simulink model "EV_Modeling"  (R2022a)
settings: Solver=FixedStepAuto  StartTime=0.0  StopTime=23612  FixedStep=0.1  RelTol=1e-3
values from neighbouring files (symbols this model uses):
  battery_SOC_SOC = battery_SOC(:,1)    [simulink.m]
  battery_SOC_voltage = battery_SOC(:,2)    [simulink.m]
  electric_consumption_ressistancce = electric_consumption(:,2)    [simulink.m]
  electric_consumption_voltage = electric_consumption(:,1)    [simulink.m]
  motor_efficiency_efficiency = table2array(motor_efficiency(2:height(motor_efficiency),2:width(motor_efficiency)))    [simulink.m]
  motor_efficiency_RPM = table2array(motor_efficiency(2:height(motor_efficiency),1))    [simulink.m]
  motor_efficiency_torque = transpose(motor_efficiency_torque)    [simulink.m]
  motor_RPM_torque = table2array(motor_torque(1:14,1))    [simulink.m]
  motor_torque_RPM = table2array(motor_torque(1:14,2))    [simulink.m]
libraries: simulink x4, simulink_extras x1, slpidlib x1
settings Model: Creator=Administrator  LastModifiedBy=jm538
settings SolverCC: AlgebraicLoopSolver=TrustRegion
settings DataIOCC: ExternalInput=EV_ModelingScenario.getElement('Input')  LoadExternalInput=on
settings DebuggingCC: UnconnectedInputMsg=warning  UnconnectedOutputMsg=warning  UnconnectedLineMsg=warning  SFMachineParentedDataDiag=warning
settings RTWCC: DLArmComputeVersion=19.05

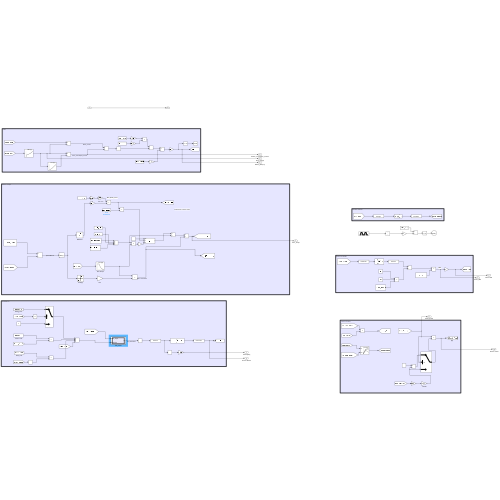
[thumbnail: Simulink's stored preview of the top-level diagram]
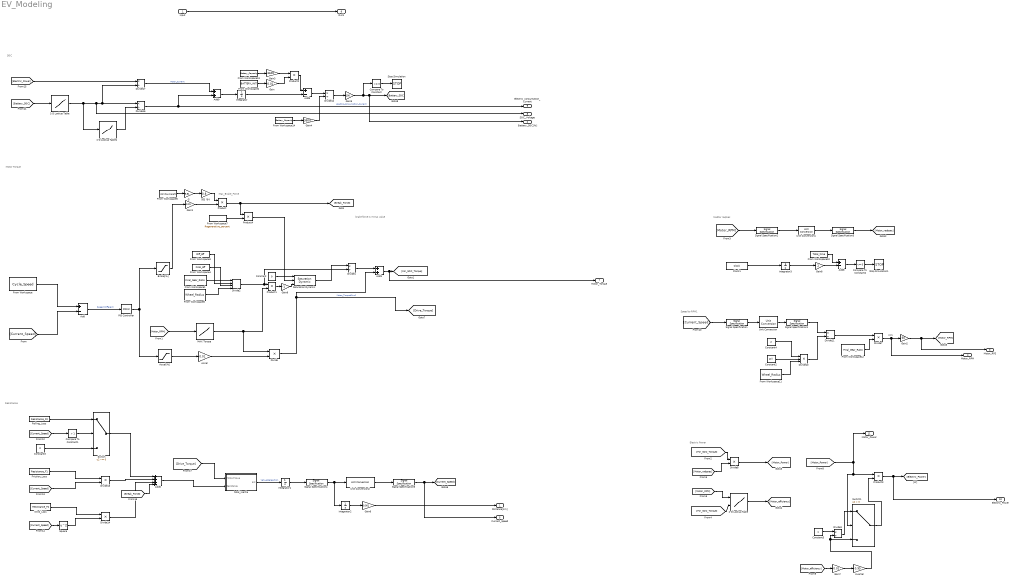
== system EV_Modeling ==
  note: brake force is minus value
  note: SOC
  note: Speed to RPM1
  note: Electric Power
  note: Resistance
  note: Motor Torque
  note: Modtor rad/sec
  note: Max_Brake_Force
  note: RPS
  Input : Inport
  1-D Lookup Table : Lookup_n-D  NumberOfTableDimensions=1  BreakpointsForDimension1=battery_SOC_SOC  Table=battery_SOC_voltage  InternalRulePriority=Speed  RndMeth=Simplest
  1-D Lookup Table1 : Lookup_n-D  NumberOfTableDimensions=1  BreakpointsForDimension1=electric_consumption_voltage  Table=electric_consumption_ressistancce  InternalRulePriority=Speed  RndMeth=Simplest
  2-D Lookup Table : Lookup_n-D  BreakpointsForDimension1=motor_efficiency_RPM  BreakpointsForDimension2=motor_efficiency_torque  Table=motor_efficiency_efficiency  InternalRulePriority=Speed  RndMeth=Simplest
      settings: InputPortMap=u0,u1
  Accel : Gain  Gain=0.01
  Accel[%] : Saturate  UpperLimit=100  LowerLimit=0
  Add : Sum  Inputs=+-
  Add1 : Sum
  Add5 : Sum  Inputs=+-
  Add6 : Sum  Inputs=+++-
  Add8 : Sum  Inputs=+-
  Add9 : Sum
  Brake[%] : Saturate  UpperLimit=0  LowerLimit=-100
  Clock1 : simulink_extras/Flip Flops/Clock  period=2
  Compare To Constant : simulink/Logic and Bit Operations/Compare To Constant  relop=<=  const=0  OutDataTypeStr=boolean
  Compare To Constant1 : simulink/Logic and Bit Operations/Compare To Constant  relop=>  const=1  OutDataTypeStr=boolean
  Compare To Constant2 : simulink/Logic and Bit Operations/Compare To Constant  relop=<=  const=0  OutDataTypeStr=boolean
  Constant : Constant  Value=0
  Constant2 : Constant  Value=pi()
  Constant3 : Constant  Value=0
  Constant4 : Constant  Value=2
  Constant5 : Constant
  Divide{,7..8,13..14} (5 alike) : Product  Inputs=**
  Divide{1,3,11..12,16..17} (6 alike) : Product  Inputs=*/
  Divide10 : Product  Inputs=***
  Divide2 : Product  Inputs=***/
  Friction_Loss : FromWorkspace  VariableName=Resistance_F1
  From Workspace : FromWorkspace  VariableName=Cycle_Speed
  From Workspace1 : FromWorkspace  VariableName=Final_Gear_Ratio
  From Workspace10 : FromWorkspace  VariableName=Total_time
  From Workspace11 : FromWorkspace  VariableName=Wheel_Radius
  From Workspace12 : FromWorkspace  VariableName=Final_Gear_Ratio
  From Workspace13 : FromWorkspace  VariableName=Battery_Capacity
  From Workspace14 : FromWorkspace  VariableName=Battery_Capacity
  From Workspace2 : FromWorkspace  VariableName=BATTERY_INIT
  From Workspace3 : FromWorkspace  VariableName=Diff_Eff
  From Workspace4 : FromWorkspace  VariableName=Final_Eff
  From Workspace5 : FromWorkspace  VariableName=Vehicle_Weight
  From Workspace6 : FromWorkspace  VariableName=Wheel_Radius
  From Workspace7 : FromWorkspace  VariableName=Regenerative_percent
  G : Gain  Gain=9.81
  Gain : Gain  Gain=0.01
  Gain1 : Gain  Gain=0.01
  Gain2 : Gain  Gain=60
  Gain3 : Gain  Gain=3600
  Gain4 : Gain  Gain=3600
  Gain5 : Gain  Gain=100
  Gain6 : Gain  Gain=0.001
  Gain7 : Gain  Gain=0.01
  Gain8 : Gain  Gain=2
  Gain9 : Gain  Gain=-1
  Integrator{,1..3} (4 alike) : Integrator
  MAX Torque : Lookup_n-D  NumberOfTableDimensions=1  BreakpointsForDimension1=motor_RPM_torque  Table=motor_torque_RPM  InternalRulePriority=Speed  RndMeth=Simplest
  PID Controller : slpidlib/PID Controller  Controller=PID  Form=Parallel  TimeDomain=Continuous-time  UseExternalTs=off  SampleTime=-1  IntegratorMethod=Forward Euler  FilterMethod=Forward Euler  ControllerParametersSource=internal  P=25  I=0.01  UseKiTs=off  D=0.0001  N=10  UseFilter=on  TunerSelectOption=Transfer Function Based (PID Tuner App)  InitialConditionSource=internal  InitialConditionForIntegrator=0  InitialConditionForFilter=0  DifferentiatorICPrevScaledInput=0  ExternalReset=none  TrackingMode=off  Kt=1  LimitOutput=off  SatLimitsSource=internal  UpperSaturationLimit=inf  LowerSaturationLimit=-inf  LinearizeAsGain=on  AntiWindupMode=none  Kb=1  POutMin=[]  POutMax=[]  IOutMin=[]  IOutMax=[]  DOutMin=[]  DOutMax=[]  NOutMin=[]  NOutMax=[]  SumOutMin=[]  SumOutMax=[]  SaturationOutMin=[]  SaturationOutMax=[]  PParamMin=[]  PParamMax=[]  IParamMin=[]  IParamMax=[]  DParamMin=[]  DParamMax=[]  NParamMin=[]  NParamMax=[]  KbParamMin=[]  KbParamMax=[]  KtParamMin=[]  KtParamMax=[]  KbOutMin=[]  KbOutMax=[]  KtOutMin=[]  KtOutMax=[]  IntegratorOutMin=[]  IntegratorOutMax=[]  FilterOutMin=[]  FilterOutMax=[]  SumI1OutMin=[]  SumI1OutMax=[]  SumI2OutMin=[]  SumI2OutMax=[]  SumI3OutMin=[]  SumI3OutMax=[]  SumI4OutMin=[]  SumI4OutMax=[]  SumDOutMin=[]  SumDOutMax=[]  DifferentiatorOutMin=[]  DifferentiatorOutMax=[]  FilterDiffOutCoefMin=[]  FilterDiffOutCoefMax=[]  ReciprocalOutMin=[]  ReciprocalOutMax=[]  SumDenOutMin=[]  SumDenOutMax=[]  SumNumOutMin=[]  SumNumOutMax=[]  DivideOutMin=[]  DivideOutMax=[]  UdiffTsProdOutMin=[]  UdiffTsProdOutMax=[]  NTsProdOutMin=[]  NTsProdOutMax=[]  UintegralTsProdOutMin=[]  UintegralTsProdOutMax=[]  UngainTsProdOutMin=[]  UngainTsProdOutMax=[]  IntegratorContinuousStateAttributes=''  IntegratorStateMustResolveToSignalObject=off  IntegratorRTWStateStorageClass=Auto  FilterContinuousStateAttributes=''  FilterStateMustResolveToSignalObject=off  FilterRTWStateStorageClass=Auto  ParallelPVariant=InternalParameters  IdealPVariant=Disabled  IVariant=InternalParameters  DVariant=InternalParameters  IntegratorVariant=Continuous  SatVariant=Disabled  AWVariant=Passthrough  PCopyVariant=Disabled  TRVariant=Disabled  FdbkBlocksVariant=Forward  IdealPFdbkVariant=Disabled  SatFdbkVariant=Disabled  DerivativeFilterVariant=ContFilter  NVariant=InternalParameters  NCopyVariant=Disabled  FilterICVariant=InternalICsFilter  IntegratorICVariant=InternalICs  ExternalResetVariant=Disabled  TRSumVariant=Passthrough  SumFdbkVariant=Disabled  SumVariant=Sum_PID  TsampFilterVariant=InternalTs  TsampNgainVariant=Passthrough  TsampIntegralVariant=Passthrough  ExternalSaturationOutDataTypeStr=Inherit: Same as second input  aMode=0
  Product{,1..4} (5 alike) : Product
  Rolling_Loss : FromWorkspace  VariableName=Resistance_F0
  Saturation Dynamic : simulink/Discontinuities/Saturation Dynamic  OutMin=[]  OutMax=[]  OutDataTypeStr=Inherit: Same as second input  OutDataType=fixdt(1, 16)  OutScaling=2^-10  DoSatur=off
  Signal Specification : SignalSpecification  Unit=km/hr
  Signal Specification1 : SignalSpecification  Unit=m/s
  Signal Specification2 : SignalSpecification  Unit=rpm
  Signal Specification3 : SignalSpecification  Unit=rad/s
  Signal Specification4 : SignalSpecification  Unit=m/s
  Signal Specification5 : SignalSpecification  Unit=km/hr
  Square : Math  Operator=square
  Stop Simulation : Stop
  Stop Simulation1 : Stop
  Switch : Switch  Criteria=u2 ~= 0  SaturateOnIntegerOverflow=off  InputSameDT=off
  Switch1 : Switch  Criteria=u2 > Threshold  SaturateOnIntegerOverflow=off  InputSameDT=off
  Unit Conversion : UnitConversion
  Unit Conversion1 : UnitConversion
  Unit Conversion2 : UnitConversion
  Wind_Loss : FromWorkspace  VariableName=Resistance_F2
  inverter : Gain  Gain=0.95
  total_inertia : Subsystem
  마찰 계수 : Gain  Gain=0.8
  Distance[km] : Outport
  Battery_SOC[%] : Outport  Port=2
  Motor_RPS : Outport  Port=3
  Motor_RPM : Outport  Port=4
  Current_Speed : Outport  Port=5
  Out1 : Outport  Port=6
  Motor_Torque : Outport  Port=7
  SOC_Voltage : Outport  Port=8
  Electric_consumption_Current : Outport  Port=9
  Electric_Power : Outport  Port=10
  Motor_Power : Outport  Port=11
  wires:
  Gain5/1 -> Battery_SOC[%]/1, [Battery_SOC], Compare To Constant/1
  1-D Lookup Table/1 -> Divide16/1, Divide17/2, SOC_Voltage/1, 1-D Lookup Table1/1
  Product3/1 -> Electric_Power/1, [Electric_Power]
  Gain6/1 -> Distance[km]/1
  Integrator3/1 -> Gain8/1
  Signal Specification5/1 -> Current_Speed/1, [Current_Speed]
  Compare To Constant2/1 -> Stop Simulation1/1
  Add8/1 -> Compare To Constant2/1
  Gain8/1 -> Add8/2
  From Workspace10/1 -> Add8/1
  Clock1/1 -> Integrator3/1
  Input/1 -> Out1/1
  Signal Specification2/1 -> Unit Conversion1/1
  Unit Conversion1/1 -> Signal Specification3/1
  Signal Specification3/1 -> [Motor_radpsec]
  Add1/1 -> Motor_Torque/1, [For_SOC_Torque]
  Divide1/1 -> Add1/1
  Divide2/1 -> Divide1/2, Product1/1
  From Workspace1/1 -> Divide2/1
  마찰 계수/1 -> Product/1
  G/1 -> 마찰 계수/1
  From Workspace5/1 -> G/1
  Accel/1 -> Divide/2
  Brake[%]/1 -> Gain1/1
  Divide/1 -> Add1/2, [Drive_Torque]  "Motor_Torque[N.m]"
  [Current_Speed] -> Add/2
  PID Controller/1 -> Brake[%]/1, Accel[%]/1
  Gain1/1 -> Product/2
  [Motor_RPM] -> MAX Torque/1
  MAX Torque/1 -> Product1/2, Divide/1
  From Workspace/1 -> Add/1
  Add/1 -> PID Controller/1  "Speed Different"
  Accel[%]/1 -> Accel/1
  [Current_Speed] -> Square/1
  Integrator2/1 -> Gain6/1
  Divide14/1 -> Add6/3
  Integrator1/1 -> Signal Specification4/1
  Wind_Loss/1 -> Divide14/1
  Signal Specification4/1 -> Integrator2/1, Unit Conversion2/1
  Unit Conversion2/1 -> Signal Specification5/1
  Rolling_Loss/1 -> Switch/1
  [Current_Speed] -> Divide13/2
  Square/1 -> Divide14/2
  total_inertia/1(acc) -> Integrator1/1  "Veh_acceleartion"
  [Current_Speed] -> Compare To Constant1/1
  Friction_Loss/1 -> Divide13/1
  Compare To Constant1/1 -> Switch/2
  Divide13/1 -> Add6/2
  Constant3/1 -> Switch/3
  Switch/1 -> Add6/1
  [Motor_RPM] -> Signal Specification2/1
  [Motor_efficiency] -> Gain7/1
  2-D Lookup Table/1 -> [Motor_efficiency]
  [For_SOC_Torque] -> Divide8/1
  [Motor_radpsec] -> Divide8/2
  Divide8/1 -> [Motor_Power]
  [For_SOC_Torque] -> 2-D Lookup Table/2
  [Motor_RPM] -> 2-D Lookup Table/1
  [Motor_Power] -> Motor_Power/1, Switch1/2, Product3/1
  From Workspace12/1 -> Divide7/2
  Constant4/1 -> Divide10/1
  Divide11/1 -> Divide7/1
  Constant2/1 -> Divide10/2
  Signal Specification1/1 -> Divide11/1
  [Current_Speed] -> Signal Specification/1
  From Workspace11/1 -> Divide10/3
  Signal Specification/1 -> Unit Conversion/1
  Gain2/1 -> Motor_RPS/1, [Motor_RPM]
  Divide10/1 -> Divide11/2
  Unit Conversion/1 -> Signal Specification1/1
  Divide7/1 -> Motor_RPM/1, Gain2/1
  Divide17/1 -> Add9/1  "Motor_Current"
  Divide12/1 -> Gain5/1
  From Workspace13/1 -> Gain3/1
  Divide16/1 -> Add9/2, Electric_consumption_Current/1  "electric_consumption_Current"
  From Workspace14/1 -> Gain4/1
  Integrator/1 -> Add5/2
  1-D Lookup Table1/1 -> Divide16/2
  [Battery_SOC] -> 1-D Lookup Table/1
  Compare To Constant/1 -> Stop Simulation/1
  Add5/1 -> Divide12/1
  Add9/1 -> Integrator/1
  [Electric_Power] -> Divide17/1
  Gain4/1 -> Divide12/2
  Product/1 -> [Break_Force], Product4/1
  [Drive_Torque] -> total_inertia/1(Motor_Toque)
  [Break_Force] -> Add6/4
  Add6/1 -> total_inertia/2(Resistance)
  From Workspace2/1 -> Gain/1
  Gain3/1 -> Product2/1
  Gain/1 -> Product2/2
  Product2/1 -> Add5/1
  Gain7/1 -> inverter/1
  Constant5/1 -> Divide3/1
  Switch1/1 -> Product3/2
  Divide3/1 -> Switch1/1
  From Workspace6/1 -> Divide2/4
  From Workspace4/1 -> Divide2/3
  From Workspace3/1 -> Divide2/2
  Product1/1 -> Gain9/1
  Gain9/1 -> Saturation Dynamic/3
  Constant/1 -> Saturation Dynamic/1
  Saturation Dynamic/1 -> Divide1/1
  From Workspace7/1 -> Product4/2
  Product4/1 -> Saturation Dynamic/2
  inverter/1 -> Divide3/2, Switch1/3

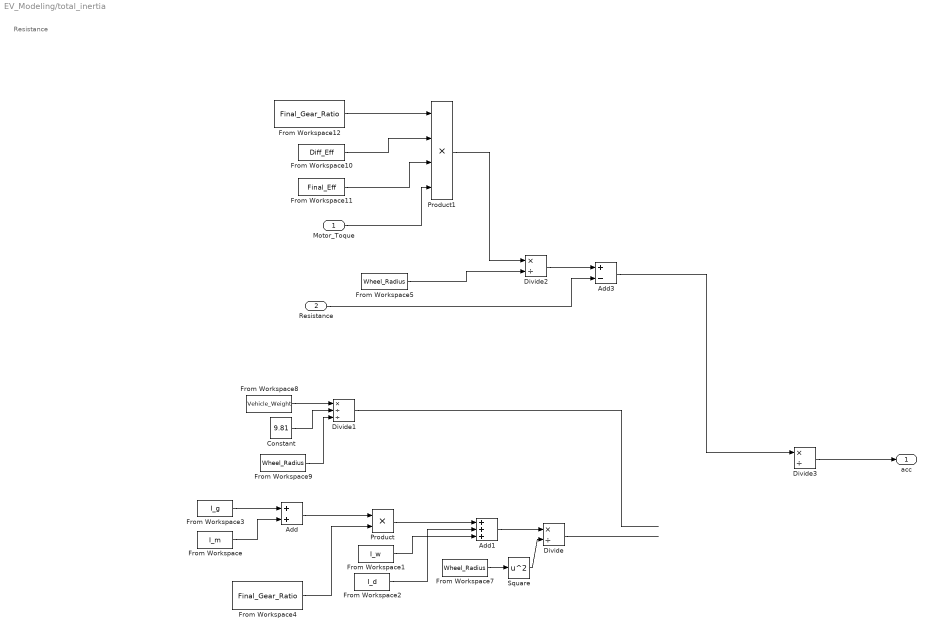
== system EV_Modeling/total_inertia ==
  note: Resistance
  Motor_Toque : Inport
  Resistance : Inport  Port=2
  Add : Sum
  Add1 : Sum  Inputs=+++
  Add3 : Sum  Inputs=+-
  Constant : Constant  Value=9.81
  Divide : Product  Inputs=*/
  Divide1 : Product  Inputs=*//
  Divide2 : Product  Inputs=*/
  Divide3 : Product  Inputs=*/
  From Workspace : FromWorkspace  VariableName=I_m
  From Workspace1 : FromWorkspace  VariableName=I_w
  From Workspace10 : FromWorkspace  VariableName=Diff_Eff
  From Workspace11 : FromWorkspace  VariableName=Final_Eff
  From Workspace12 : FromWorkspace  VariableName=Final_Gear_Ratio
  From Workspace2 : FromWorkspace  VariableName=I_d
  From Workspace3 : FromWorkspace  VariableName=I_g
  From Workspace4 : FromWorkspace  VariableName=Final_Gear_Ratio
  From Workspace5 : FromWorkspace  VariableName=Wheel_Radius
  From Workspace7 : FromWorkspace  VariableName=Wheel_Radius
  From Workspace8 : FromWorkspace  VariableName=Vehicle_Weight
  From Workspace9 : FromWorkspace  VariableName=Wheel_Radius
  Product : Product
  Product1 : Product  Inputs=4
  Square : Math  Operator=square
  acc : Outport
  wires:
  Divide3/1 -> acc/1
  From Workspace7/1 -> Square/1
  From Workspace9/1 -> Divide1/3
  ? -> Divide3/2
  From Workspace8/1 -> Divide1/1
  Resistance/1 -> Add3/2
  From Workspace4/1 -> Product/2
  Square/1 -> Divide/2
  Add/1 -> Product/1
  From Workspace3/1 -> Add/1
  Divide1/1 -> ?
  From Workspace/1 -> Add/2
  Divide2/1 -> Add3/1
  From Workspace1/1 -> Add1/3
  From Workspace2/1 -> Add1/2
  Product/1 -> Add1/1
  Divide/1 -> ?
  Add1/1 -> Divide/1
  Constant/1 -> Divide1/2
  Add3/1 -> Divide3/1
  From Workspace12/1 -> Product1/1
  From Workspace10/1 -> Product1/2
  From Workspace11/1 -> Product1/3
  Motor_Toque/1 -> Product1/4
  Product1/1 -> Divide2/1
  From Workspace5/1 -> Divide2/2
